simulink model "CSTRExample"  (R2020a)
settings: Solver=VariableStepAuto  StartTime=0.0  StopTime=20  MaxStep=100e-3  RelTol=1e-3
settings Model: Creator=david  LastModifiedBy=david

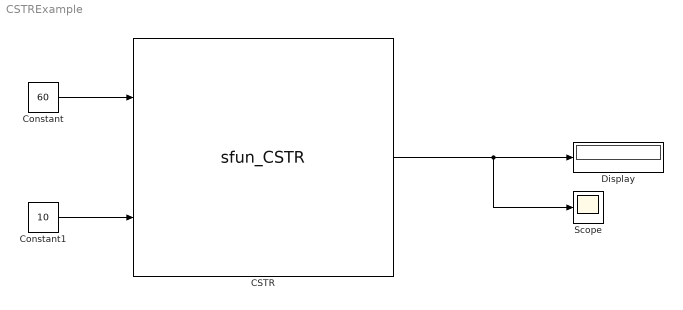
== system CSTRExample ==
  CSTR : M-S-Function  FunctionName=sfun_CSTR  Parameters=|  mask{k1=5/6, k2=5/3, k3=1/6, V=700, Ca0=2.9175, Cb0=1.10}
      | [k1;
      | k2;
      | k3; V], [Ca0; Cb0]
      mask DialogControl DescGroupVar Prompt: CSTR
      mask DialogControl DescTextVar Prompt: Isothermal CSTR with Van de Vusse dynamics
      mask Display:
      | port_label('input',1,'u');
      | port_label('input',2,'Cai');
      | port_label('output',1,'y');
      | image('VandeVusse.png')
  Constant : Constant  Value=60
  Constant1 : Constant  Value=10
  Display : Display
  Scope : Scope
  wires:
  Constant/1 -> CSTR/1
  Constant1/1 -> CSTR/2
  CSTR/1 -> Scope/1, Display/1
